simulink model "C_to_F"  (R2025b)
settings: Solver=VariableStepAuto  StartTime=0.0  StopTime=10.0  RelTol=1e-3
settings Model: Creator=ryana  LastModifiedBy=ryana

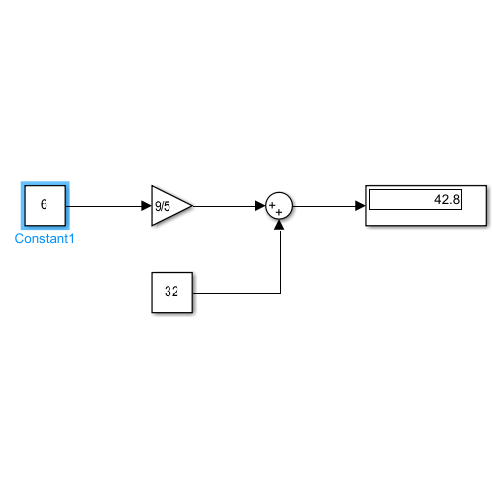
[thumbnail: Simulink's stored preview of the top-level diagram]
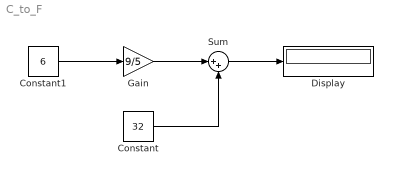
== system C_to_F ==
  Constant : Constant  Value=32
  Constant1 : Constant  Value=6
  Display : Display
  Gain : Gain  Gain=9/5
  Sum : Sum  Inputs=|++
  wires:
  Gain/1 -> Sum/1
  Constant/1 -> Sum/2
  Sum/1 -> Display/1
  Constant1/1 -> Gain/1
